simulink model "addANDaccum1"  (R2024b)
settings: Solver=FixedStepAuto  StartTime=0.0  StopTime=10.0  FixedStep=1  RelTol=1e-3  EnableMultiTasking=on
settings Model: Creator=shan2  LastModifiedBy=marmar
settings SolverCC: AlgebraicLoopSolver=TrustRegion
settings DataIOCC: LimitDataPoints=on  SaveFormat=Array  ReturnWorkspaceOutputs=off
settings OptimizationCC: LifeSpan=inf
settings DebuggingCC: SolverPrmCheckMsg=warning  UnconnectedInputMsg=warning  UnconnectedOutputMsg=warning  UnconnectedLineMsg=warning  SFUnexpectedBacktrackingDiag=warning  SFNoUnconditionalDefaultTransitionDiag=warning  SFExecutionAtInitializationDiag=none  ArithmeticOperatorsInVariantConditions=warning
settings HardwareCC: ProdBitPerPointer=32  ProdBitPerSizeT=32  ProdBitPerPtrDiffT=32  ProdLargestAtomicFloat=None  ProdIntDivRoundTo=Undefined  ProdEndianess=Unspecified  ProdWordSize=32  ProdHWDeviceType=32-bit Generic
settings ModelReferenceCC: PropagateSignalLabelsOutOfModel=off
settings SFSimCC: SimUseLocalCustomCode=off  CustomCodeUndefinedFunction=UseInterfaceOnly
settings RTWCC: RTWUseLocalCustomCode=off  GPUComputeCapability=3.5
settings CodeAppCC: StateflowObjectComments=on
settings GRTTargetCC: TargetLangStandard=C89/C90 (ANSI)
settings ConfigComp: CovMetricSettings=dw  CovSaveCumulativeToWorkspaceVar=on  CovSaveSingleToWorkspaceVar=on  CovExternalEMLEnable=off  CovSFcnEnable=off

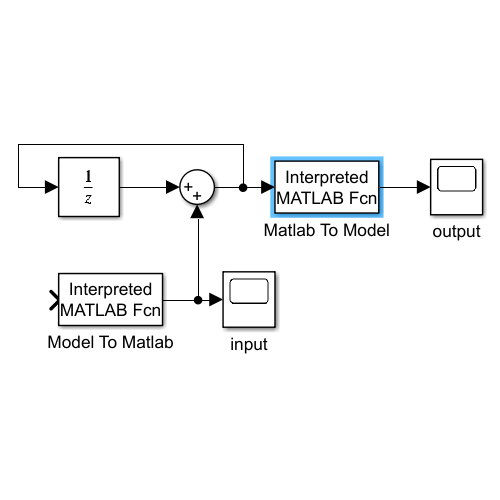
[thumbnail: Simulink's stored preview of the top-level diagram]
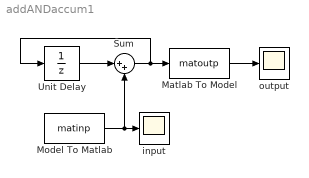
== system addANDaccum1 ==
  Matlab To Model : MATLABFcn  StartFcn=|  StopFcn=evalin('base','fclose(fidout);');  MATLABFcn=matoutp  OutputDimensions=1
      | evalin('base','fidout = fopen(''addANDaccum1_out'',''w'');');
      | %fprintf(evalin('base','fidout'),'0\n0\n0\n');
  Model To Matlab : MATLABFcn  StartFcn=evalin('base','fidin = fopen(''addANDaccum1_inp'',''r'');');  StopFcn=evalin('base','fclose(fidin);');  MATLABFcn=matinp  OutputDimensions=1
  Sum : Sum  Inputs=|++
  Unit Delay : UnitDelay  HasFrameUpgradeWarning=on
  input : Scope
  output : Scope
  wires:
  Sum/1 -> Matlab To Model/1, Unit Delay/1
  Unit Delay/1 -> Sum/1
  Model To Matlab/1 -> input/1, Sum/2
  Matlab To Model/1 -> output/1
